simulink model "B3"  (R2023a)
settings: Solver=VariableStepAuto  StartTime=0.0  StopTime=1  RelTol=1e-3
undefined symbols (not defined in the file): K, L, omega
settings Model: Creator=86173  LastModifiedBy=86173

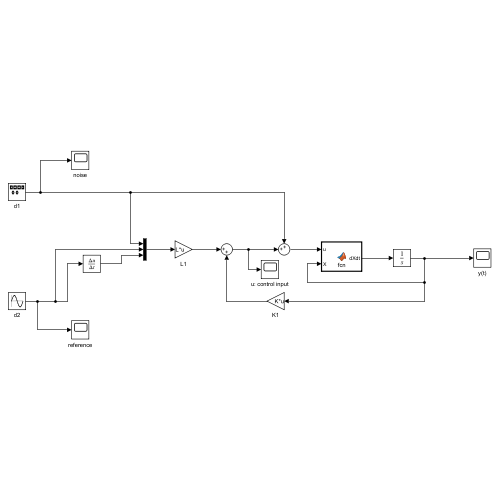
[thumbnail: Simulink's stored preview of the top-level diagram]
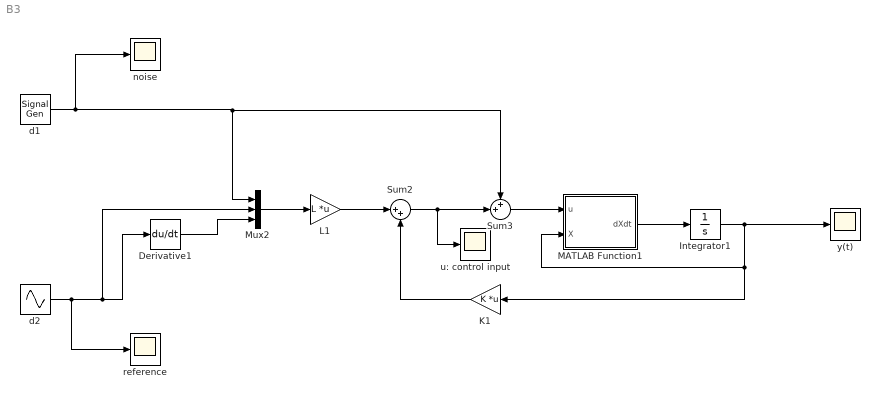
== system B3 ==
  Derivative1 : Derivative
  Integrator1 : Integrator  InitialCondition=[0,0,0,0]
  K1 : Gain  Gain=K  Multiplication=Matrix(K*u)
  L1 : Gain  Gain=L  Multiplication=Matrix(K*u)
  MATLAB Function1 : MATLAB Function  TreatAsAtomicUnit=on
  Mux2 : Mux  Inputs=3
  Sum2 : Sum  Inputs=|++
  Sum3 : Sum  Inputs=++|
  d1 : SignalGenerator  WaveForm=square  Amplitude=0.5  Frequency=0.02
  d2 : Sin  Frequency=omega  SampleTime=0
  noise : Scope
  reference : Scope
  u: control input : Scope
  y(t) : Scope
  wires:
  Sum2/1 -> u: control input/1, Sum3/2
  Mux2/1 -> L1/1
  d1/1 -> noise/1, Sum3/1, Mux2/1
  K1/1 -> Sum2/2
  d2/1 -> reference/1, Derivative1/1, Mux2/2
  L1/1 -> Sum2/1
  Derivative1/1 -> Mux2/3
  Sum3/1 -> MATLAB Function1/1("u ")
  MATLAB Function1/1(dXdt) -> Integrator1/1
  Integrator1/1 -> y(t)/1, MATLAB Function1/2(X), K1/1

== matlab function B3/MATLAB Function1 ==
  data: u input; dXdt output; X input
function dXdt =  fcn(u,X)

    x1 = X(1); % s
    x2 = X(2); % s_dot
    x3 = X(3); % phi
    x4 = X(4); % phi_dot
    
    % system dynamics
    dx1 = x2;
    dx2 = -1*x2 + u; % 在这里 u d 已经合并了
    dx3 = x4;
    dx4 = -1*(-1*x2 + u)*cos(x3) + 9.81*sin(x3);

    dXdt = [dx1; dx2; dx3; dx4];

end
